simulink model "IEEE34_PMSG"  (R2024a)
settings: Solver=FixedStepDiscrete  StartTime=0.0  StopTime=ttotal  RelTol=1e-3
values from neighbouring files (symbols this model uses):
  C0_300 = 4.9597e-09    [Data_input_DFIG.mat]    (also in Data_input_PMSG.mat)
  C0_301 = 4.8339e-09    [Data_input_DFIG.mat]    (also in Data_input_PMSG.mat)
  C1_300 = 1.0146e-08    [Data_input_DFIG.mat]    (also in Data_input_PMSG.mat)
  C1_301 = 9.7319e-09    [Data_input_DFIG.mat]    (also in Data_input_PMSG.mat)
  CC = [20000 9000 135000 20000 150000 10000 16000 7000 105000 16000 75000 5000 ... (36 elements, 6x6)]    [Data_input_DFIG.mat]    (also in Data_input_PMSG.mat)
  CD = [0 0 34000 135000 0 0 0 7000 0 7000 2000 4000 ... (114 elements, 19x6)]    [Data_input_DFIG.mat]    (also in Data_input_PMSG.mat)
  cte = 1e-06    [Data_input_DFIG.mat]    (also in Data_input_PMSG.mat)
  L0_300 = 0.0039    [Data_input_DFIG.mat]    (also in Data_input_PMSG.mat)
  L0_301 = 0.0043    [Data_input_DFIG.mat]    (also in Data_input_PMSG.mat)
  L1_300 = 0.0014    [Data_input_DFIG.mat]    (also in Data_input_PMSG.mat)
  L1_301 = 0.0014    [Data_input_DFIG.mat]    (also in Data_input_PMSG.mat)
  R0_300 = 1.0909    [Data_input_DFIG.mat]    (also in Data_input_PMSG.mat)
  R0_301 = 1.4885    [Data_input_DFIG.mat]    (also in Data_input_PMSG.mat)
  R1_300 = 0.6983    [Data_input_DFIG.mat]    (also in Data_input_PMSG.mat)
  R1_301 = 1.0537    [Data_input_DFIG.mat]    (also in Data_input_PMSG.mat)
  tf_AB = 1.75    [Data_input_DFIG.mat]    (also in Data_input_PMSG.mat = 2.65)
  tf_ABC = 1.75    [Data_input_DFIG.mat]    (also in Data_input_PMSG.mat = 2.65)
  tf_ABT = 1.75    [Data_input_DFIG.mat]    (also in Data_input_PMSG.mat = 2.65)
  tf_AT = 1.75    [Data_input_DFIG.mat]    (also in Data_input_PMSG.mat = 2.65)
  tf_BC = 1.75    [Data_input_DFIG.mat]    (also in Data_input_PMSG.mat = 2.65)
  tf_BCT = 1.75    [Data_input_DFIG.mat]    (also in Data_input_PMSG.mat = 2.65)
  tf_BT = 1.75    [Data_input_DFIG.mat]    (also in Data_input_PMSG.mat = 2.65)
  tf_CA = 1.75    [Data_input_DFIG.mat]    (also in Data_input_PMSG.mat = 2.65)
  tf_CAT = 1.75    [Data_input_DFIG.mat]    (also in Data_input_PMSG.mat = 2.65)
  tf_CT = 1.75    [Data_input_DFIG.mat]    (also in Data_input_PMSG.mat = 2.65)
  Ts = 5.008e-06    [Data_input_DFIG.mat]    (also in Data_input_PMSG.mat = 1.0016e-05)
undefined symbols (not defined in the file or in its folder): D1, Delta, DiscIntNeverNeededParam, find_system
libraries: spsThreePhaseSeriesRLCLoadLib x31, spsThreePhasePISectionLineLib x22, spsGroundLib x15, spsSeriesRLCLoadLib x14, spsThreePhaseFaultLib x10, spsSecondOrderFilterLib x9, spsPiSectionLineLib x8, spsThreePhaseVIMeasurementLib x6, spsabctodq0Lib x5, simulink_extras x4, spsFirstOrderFilterLib x4, spsThreePhaseTransformerTwoWindingsLib x3
(part 1 of 4)
settings Model: Creator=hani  LastModifiedBy=jucar
settings SolverCC: AlgebraicLoopSolver=TrustRegion
settings DataIOCC: LimitDataPoints=on  SaveFormat=Array  SignalLoggingSaveFormat=ModelDataLogs  ReturnWorkspaceOutputs=off
settings OptimizationCC: ExpressionDepthLimit=2147483647  LifeSpan=inf
settings DebuggingCC: UnderspecifiedInitializationDetection=Classic  MergeDetectMultiDrivingBlocksExec=none  FcnCallInpInsideContextMsg=warning  UnconnectedInputMsg=warning  UnconnectedOutputMsg=warning  UnconnectedLineMsg=warning  StateNameClashWarn=warning  SFUnexpectedBacktrackingDiag=warning  SFNoUnconditionalDefaultTransitionDiag=warning  SFExecutionAtInitializationDiag=none  ArithmeticOperatorsInVariantConditions=warning
settings HardwareCC: ProdBitPerPointer=32  ProdBitPerSizeT=32  ProdBitPerPtrDiffT=32  ProdLargestAtomicFloat=None  ProdIntDivRoundTo=Undefined  ProdEndianess=Unspecified  ProdWordSize=32  ProdHWDeviceType=32-bit Generic
settings ModelReferenceCC: EnableRefExpFcnMdlSchedulingChecks=on  PropagateSignalLabelsOutOfModel=off
settings SFSimCC: SimUseLocalCustomCode=off  SimParseCustomCode=off  CustomCodeUndefinedFunction=UseInterfaceOnly
settings RTWCC: RTWUseLocalCustomCode=off  GPUComputeCapability=3.5
settings CodeAppCC: StateflowObjectComments=on
settings GRTTargetCC: TargetLangStandard=C89/C90 (ANSI)  CombineOutputUpdateFcns=off  GRTInterface=on
settings ConfigComp: CovMetricSettings=dw  CovSaveCumulativeToWorkspaceVar=on  CovSaveSingleToWorkspaceVar=on  CovExternalEMLEnable=off

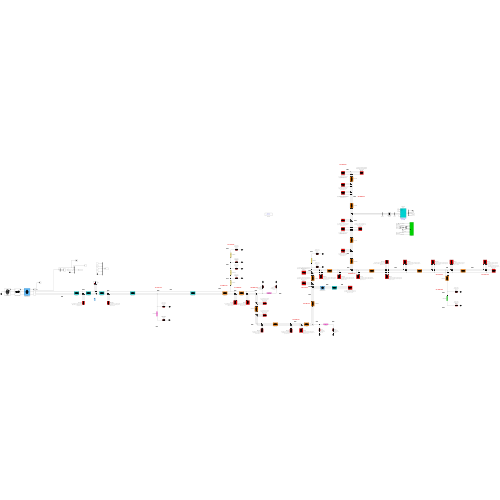
[thumbnail: Simulink's stored preview of the top-level diagram]
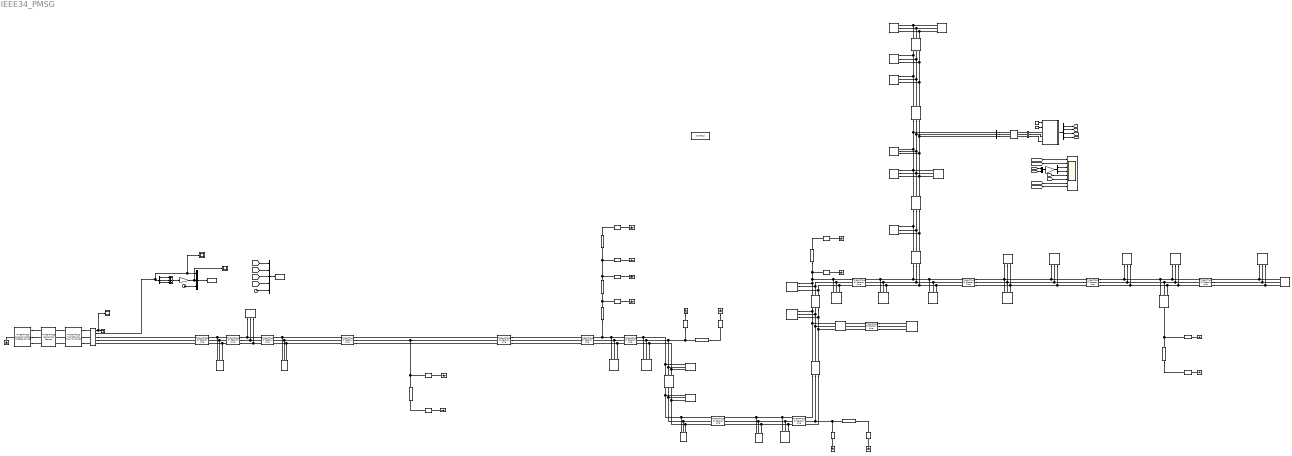
== system IEEE34_PMSG ==
  note: 806
  note: 832
  note: 862
  note: 842
  note: 808
  note: 800
  note: 826
  note: 844
  note: 850
  note: 834
  note: 830
  note: 824
  note: 848
  note: 840
  note: 838
  note: 888
  note: 854
  note: 57.5888 km
  note: 858
  note: 846
  note: 41.3247 km
  note: 864
  note: 890
  note: 816
  note: 860
  note: 856
  note: 55.9825 km
  note: 31.6291 km
  note: 57.7503 km
  note: 802
  note: 828
  note: 11.1374 km
  note: 34.8386 km
  note: 836
  note: 52.709 km
  note: 52.712 km
  note: 57.6772 km
  note: 852
  note: 1
  note: 810
  note: 820
  note: 818
  note: 51.1119 km
  note: 822
  note: 31.7266 km
  note: 57.4151 km
  note: 57.5004 km
  note: 812
  note: 10 MW Wind Farm
      | (5 x 2 MW)
  " " : spsThreePhaseVIMeasurementLib/Three-Phase V-I Measurement  VoltageMeasurement=phase-to-ground  SetLabelV=off  LabelV=Vabc  Vpu=off  VpuLL=off  CurrentMeasurement=yes  SetLabelI=off  LabelI=Iabc  Ipu=off  Pbase=100e6  Vbase=24.9e3  OutputType=Complex  PhasorSimulation=off  PSBequivalent=0
  0.0853 km : spsThreePhasePISectionLineLib/Three-Phase PI Section Line  LConnTagsString=a|b|c  RConnTagsString=A|B|C  Length=0.0853  Frequency=60  Resistances=[ R1_301 R0_301]  Inductances=[ L1_301 L0_301]  Capacitances=[C1_301 C0_301]
  0.0853 km1 : spsThreePhasePISectionLineLib/Three-Phase PI Section Line  LConnTagsString=a|b|c  RConnTagsString=A|B|C  Length=0.0853  Frequency=60  Resistances=[ R1_301 R0_301]  Inductances=[ L1_301 L0_301]  Capacitances=[C1_301 C0_301]
  0.0975 km : spsThreePhasePISectionLineLib/Three-Phase PI Section Line  LConnTagsString=a|b|c  RConnTagsString=A|B|C  Length=0.0975  Frequency=60  Resistances=[ R1_301 R0_301]  Inductances=[ L1_301 L0_301]  Capacitances=[C1_301 C0_301]
  0.1585 km : spsThreePhasePISectionLineLib/Three-Phase PI Section Line  LConnTagsString=a|b|c  RConnTagsString=A|B|C  Length=0.1585  Frequency=60  Resistances=[ R1_301 R0_301]  Inductances=[ L1_301 L0_301]  Capacitances=[C1_301 C0_301]
  0.1615 km : spsThreePhasePISectionLineLib/Three-Phase PI Section Line  LConnTagsString=a|b|c  RConnTagsString=A|B|C  Length=0.1615  Frequency=60  Resistances=[ R1_301 R0_301]  Inductances=[ L1_301 L0_301]  Capacitances=[C1_301 C0_301]
  0.2136 km : spsThreePhasePISectionLineLib/Three-Phase PI Section Line  LConnTagsString=a|b|c  RConnTagsString=A|B|C  Length=0.2136  Frequency=60  Resistances=[ R1_300 R0_300]  Inductances=[ L1_300 L0_300]  Capacitances=[C1_300 C0_300]
  0.2560 km : spsThreePhasePISectionLineLib/Three-Phase PI Section Line  LConnTagsString=a|b|c  RConnTagsString=A|B|C  Length=0.2560  Frequency=60  Resistances=[ R1_301 R0_301]  Inductances=[ L1_301 L0_301]  Capacitances=[C1_301 C0_301]
  0.2621 km : spsThreePhasePISectionLineLib/Three-Phase PI Section Line  LConnTagsString=a|b|c  RConnTagsString=A|B|C  Length=0.2621  Frequency=60  Resistances=[ R1_301 R0_301]  Inductances=[ L1_301 L0_301]  Capacitances=[C1_301 C0_301]
  0.3137 km : spsThreePhasePISectionLineLib/Three-Phase PI Section Line  LConnTagsString=a|b|c  RConnTagsString=A|B|C  Length=0.3137  Frequency=60  Resistances=[ R1_300 R0_300]  Inductances=[ L1_300 L0_300]  Capacitances=[C1_300 C0_300]
  0.4115 km : spsThreePhasePISectionLineLib/Three-Phase PI Section Line  LConnTagsString=a|b|c  RConnTagsString=A|B|C  Length=0.4115  Frequency=60  Resistances=[ R1_301 R0_301]  Inductances=[ L1_301 L0_301]  Capacitances=[C1_301 C0_301]
  0.4938 Km : spsPiSectionLineLib/Pi Section Line  LConnTagsString=__new0  RConnTagsString=__new0  Phases=1  PiSections=1  Length=0.4938  Frequency=60  Resistance=1.7395  Inductance=2.4e-3  Capacitance=6.964e-9  SpecifyConductance=off  Conductance=0  Measurements=None  Measurements2=None
      settings: LibrarySourceBlock=sps_lib/Power Grid Elements/Pi Section Line
  0.5212 Km : spsPiSectionLineLib/Pi Section Line  LConnTagsString=__new0  RConnTagsString=__new0  Phases=1  PiSections=1  Length=0.5212  Frequency=60  Resistance=1.7395  Inductance=2.4e-3  Capacitance=6.964e-9  SpecifyConductance=off  Conductance=0  Measurements=None  Measurements2=None
      settings: LibrarySourceBlock=sps_lib/Power Grid Elements/Pi Section Line
  0.6157 km : spsThreePhasePISectionLineLib/Three-Phase PI Section Line  LConnTagsString=a|b|c  RConnTagsString=A|B|C  Length=0.6157  Frequency=60  Resistances=[ R1_301 R0_301]  Inductances=[ L1_301 L0_301]  Capacitances=[C1_301 C0_301]
  0.7864 km : spsThreePhasePISectionLineLib/Three-Phase PI Section Line  LConnTagsString=a|b|c  RConnTagsString=A|B|C  Length=0.7864  Frequency=60  Resistances=[ R1_300 R0_300]  Inductances=[ L1_300 L0_300]  Capacitances=[C1_300 C0_300]
  0.8169 km : spsThreePhasePISectionLineLib/Three-Phase PI Section Line  LConnTagsString=a|b|c  RConnTagsString=A|B|C  Length=0.8169  Frequency=60  Resistances=[ R1_301 R0_301]  Inductances=[ L1_301 L0_301]  Capacitances=[C1_301 C0_301]
  1.05*345 kV : spsThreePhaseProgrammableVoltageSourceLib/Three-Phase Programmable Voltage Source  PositiveSequence=[1.05*345e3 0 60]  VariationEntity=None  VariationType=Table of time-amplitude pairs  VariationTypeAlt=Step  VariationStep=0.2  VariationRate=10  VariationMagnitude=0.3  VariationFrequency=2  VariationTiming="[5  20]"  VariationPhaseA=off  Amplitudes="[ 1 0.95   1.1 ]"  TimeValues="[0  10 50]"  HarmonicGeneration=off  HarmonicA=[3 0.2 -25 0]  HarmonicB=[2 0.15 35 2]  Timing="[0.05  3]"  BusType=swing  Pref=0  Qref=0  Qmin=-inf  Qmax=inf
  1.1095 km : spsThreePhasePISectionLineLib/Three-Phase PI Section Line  LConnTagsString=a|b|c  RConnTagsString=A|B|C  Length=1.1095  Frequency=60  Resistances=[ R1_301 R0_301]  Inductances=[ L1_301 L0_301]  Capacitances=[C1_301 C0_301]
  1.4813 Km : spsPiSectionLineLib/Pi Section Line  LConnTagsString=__new0  RConnTagsString=__new0  Phases=1  PiSections=1  Length=1.4813  Frequency=60  Resistance=1.1941  Inductance=2.3e-3  Capacitance=7.1924e-9  SpecifyConductance=off  Conductance=0  Measurements=None  Measurements2=None
      settings: LibrarySourceBlock=sps_lib/Power Grid Elements/Pi Section Line
  1.4935 km : spsThreePhasePISectionLineLib/Three-Phase PI Section Line  LConnTagsString=a|b|c  RConnTagsString=A|B|C  Length=1.4935  Frequency=60  Resistances=[ R1_301 R0_301]  Inductances=[ L1_301 L0_301]  Capacitances=[C1_301 C0_301]
  1.7691 Km : spsPiSectionLineLib/Pi Section Line  LConnTagsString=__new0  RConnTagsString=__new0  Phases=1  PiSections=1  Length=1.7691  Frequency=60  Resistance=1.7395  Inductance=2.4e-3  Capacitance=6.964e-9  SpecifyConductance=off  Conductance=0  Measurements=None  Measurements2=None
      settings: LibrarySourceBlock=sps_lib/Power Grid Elements/Pi Section Line
  1.7691 Km1 : spsPiSectionLineLib/Pi Section Line  LConnTagsString=__new0  RConnTagsString=__new0  Phases=1  PiSections=1  Length=1.7691  Frequency=60  Resistance=1.7395  Inductance=2.4e-3  Capacitance=6.964e-9  SpecifyConductance=off  Conductance=0  Measurements=None  Measurements2=None
      settings: LibrarySourceBlock=sps_lib/Power Grid Elements/Pi Section Line
  1.7770 km : spsThreePhasePISectionLineLib/Three-Phase PI Section Line  LConnTagsString=a|b|c  RConnTagsString=A|B|C  Length=1.7770  Frequency=60  Resistances=[ R1_301 R0_301]  Inductances=[ L1_301 L0_301]  Capacitances=[C1_301 C0_301]
  11.2288 km : spsThreePhasePISectionLineLib/Three-Phase PI Section Line  LConnTagsString=a|b|c  RConnTagsString=A|B|C  Length=11.2288  Frequency=60  Resistances=[ R1_301 R0_301]  Inductances=[ L1_301 L0_301]  Capacitances=[C1_301 C0_301]
  14.6761 Km : spsPiSectionLineLib/Pi Section Line  LConnTagsString=__new0  RConnTagsString=__new0  Phases=1  PiSections=1  Length=14.6761  Frequency=60  Resistance=1.7395  Inductance=2.4e-3  Capacitance=6.964e-9  SpecifyConductance=off  Conductance=0  Measurements=None  Measurements2=None
      settings: LibrarySourceBlock=sps_lib/Power Grid Elements/Pi Section Line
  2.5 MVA 345 KV/24.9 KV : spsThreePhaseTransformerTwoWindingsLib/Three-Phase Transformer (Two Windings)  Winding1Connection=Delta (D1)  Winding2Connection=Yg  CoreType=Three single-phase transformers  SetSaturation=off  Hysteresis=off  DataFile='hysteresis'  SetInitialFlux=off  Measurements=None  UNITS=pu  NominalPower=[ 2500e3 , 60 ]  Winding1=[345e3, 0.01, 0.08 ]  Winding2=[24.9e3 , 0.01, 0.08 ]  Rm=500  Lm=500  L0=0.5  Saturation=[ 0,0 ; 0.0024,1.2 ; 1.0,1.52 ]  InitialFluxes=[ 0.8 , -0.8 , 0.7 ]  BreakLoop=off  DiscreteSolver=Trapezoidal iterative  DataType=off  TransfoNumber=1
  20.4917 km : spsThreePhasePISectionLineLib/Three-Phase PI Section Line  LConnTagsString=a|b|c  RConnTagsString=A|B|C  Length=20.4917  Frequency=60  Resistances=[ R1_300 R0_300]  Inductances=[ L1_300 L0_300]  Capacitances=[C1_300 C0_300]
  24.9 kV/ 575 V 1.25 MVA : spsThreePhaseTransformerTwoWindingsLib/Three-Phase Transformer (Two Windings)  Winding1Connection=Yg  Winding2Connection=Yg  CoreType=Three single-phase transformers  SetSaturation=off  Hysteresis=off  DataFile='hysteresis'  SetInitialFlux=off  Measurements=None  UNITS=pu  NominalPower="[1.25e6  60]"  Winding1=[24.9e3 , 0.025/30 , 0.025]  Winding2=[575, 0.025/30 , 0.025]  Rm=500  Lm=inf  L0=0.5  Saturation=[ 0,0 ; 0.0024,1.2 ; 1.0,1.52 ]  InitialFluxes=[ 0.8 , -0.8 , 0.7 ]  BreakLoop=off  DiscreteSolver=Trapezoidal iterative  DataType=off  TransfoNumber=0
  3.1120 km : spsThreePhasePISectionLineLib/Three-Phase PI Section Line  LConnTagsString=a|b|c  RConnTagsString=A|B|C  Length=3.1120  Frequency=60  Resistances=[ R1_301 R0_301]  Inductances=[ L1_301 L0_301]  Capacitances=[C1_301 C0_301]
  3.2187 km : spsThreePhasePISectionLineLib/Three-Phase PI Section Line  LConnTagsString=a|b|c  RConnTagsString=A|B|C  Length=3.2187  Frequency=60  Resistances=[ R1_300 R0_300]  Inductances=[ L1_300 L0_300]  Capacitances=[C1_300 C0_300]
  4.1880 Km : spsPiSectionLineLib/Pi Section Line  LConnTagsString=__new0  RConnTagsString=__new0  Phases=1  PiSections=1  Length=4.1880  Frequency=60  Resistance=1.7395  Inductance=2.4e-3  Capacitance=6.964e-9  SpecifyConductance=off  Conductance=0  Measurements=None  Measurements2=None
      settings: LibrarySourceBlock=sps_lib/Power Grid Elements/Pi Section Line
  500 kVA 24.9 KV/4.16 KV : spsThreePhaseTransformerTwoWindingsLib/Three-Phase Transformer (Two Windings)  Winding1Connection=Yg  Winding2Connection=Yg  CoreType=Three single-phase transformers  SetSaturation=off  Hysteresis=off  DataFile='hysteresis'  SetInitialFlux=off  Measurements=None  UNITS=pu  NominalPower=[ 500e3 , 60 ]  Winding1=[24.9e3 , 0.019 , 0.0408 ]  Winding2=[ 4.16e3 , 0.019 , 0.0408 ]  Rm=500  Lm=500  L0=0.5  Saturation=[ 0,0 ; 0.0024,1.2 ; 1.0,1.52 ]  InitialFluxes=[ 0.8 , -0.8 , 0.7 ]  BreakLoop=off  DiscreteSolver=Trapezoidal iterative  DataType=off  TransfoNumber=1
  6.2301 km : spsThreePhasePISectionLineLib/Three-Phase PI Section Line  LConnTagsString=a|b|c  RConnTagsString=A|B|C  Length=6.2301  Frequency=60  Resistances=[ R1_301 R0_301]  Inductances=[ L1_301 L0_301]  Capacitances=[C1_301 C0_301]
  7.1110 Km : spsPiSectionLineLib/Pi Section Line  LConnTagsString=__new0  RConnTagsString=__new0  Phases=1  PiSections=1  Length=7.1110  Frequency=60  Resistance=1.7395  Inductance=2.4e-3  Capacitance=6.964e-9  SpecifyConductance=off  Conductance=0  Measurements=None  Measurements2=None
      settings: LibrarySourceBlock=sps_lib/Power Grid Elements/Pi Section Line
  802 Yg-PQ : spsThreePhaseSeriesRLCLoadLib/Three-Phase Series RLC Load  LConnTagsString=A|B|C  Configuration=Y (grounded)  NominalVoltage=120e3  Vabc=[ 1.04738 1.04828 1.0485]*14376  Vabcp=[1e3 1e3 1e3]  NominalFrequency=60  UnbalancedPower=on  ActivePower=1e+006  InductivePower=0  CapacitivePower=0  Pabc="[cte CD(1,3)  CD(1,5)]/2"  QLabc=[0 CD(1,4) CD(1,6)]/2  QCabc=[0 0 0]  Pabcp=[10e3 9e3 11e3]  QLabcp=[100 90 110]  QCabcp=[100 90 110]  Measurements=None  LoadType=constant PQ
      settings: AttributesFormatString=|
      | P= %<Pabc> W
      | Ql=%<QLabc> var
      | Qc=%<QCabc> var
  806 Yg-PQ : spsThreePhaseSeriesRLCLoadLib/Three-Phase Series RLC Load  LConnTagsString=A|B|C  Configuration=Y (grounded)  NominalVoltage=120e3  Vabc=[ 1.04562 1.04717 1.04753]*14376  Vabcp=[1e3 1e3 1e3]  NominalFrequency=60  UnbalancedPower=on  ActivePower=1e+006  InductivePower=0  CapacitivePower=0  Pabc="[cte CD(1,3)  CD(1,5)]/2"  QLabc=[0 CD(1,4) CD(1,6)]/2  QCabc=[0 0 0]  Pabcp=[10e3 9e3 11e3]  QLabcp=[100 90 110]  QCabcp=[100 90 110]  Measurements=None  LoadType=constant PQ
      settings: AttributesFormatString=|
      | P= %<Pabc> W
      | Ql=%<QLabc> var
      | Qc=%<QCabc> var
  808-I : spsSeriesRLCLoadLib/Series RLC Load  LConnTagsString=a  RConnTagsString=__new0  NominalVoltage=1.01367*14376  NominalFrequency=60  ActivePower=CD(2,3)/2  InductivePower=CD(2,4)/2  CapacitivePower=0  Setx0=off  InitialVoltage=0  SetiL0=off  InitialCurrent=0  Measurements=None  LoadType=constant I
      settings: AttributesFormatString=|
      | P=%<ActivePower> W
      | Ql=%<InductivePower> var
      | Qc=%<CapacitivePower> var
  810-I : spsSeriesRLCLoadLib/Series RLC Load  LConnTagsString=a  RConnTagsString=__new0  NominalVoltage=1.0136*14376  NominalFrequency=60  ActivePower=CD(2,3)/2  InductivePower=CD(2,4)/2  CapacitivePower=0  Setx0=off  InitialVoltage=0  SetiL0=off  InitialCurrent=0  Measurements=None  LoadType=constant I
      settings: AttributesFormatString=|
      | P=%<ActivePower> W
      | Ql=%<InductivePower> var
      | Qc=%<CapacitivePower> var
  816 D-I : spsThreePhaseSeriesRLCLoadLib/Three-Phase Series RLC Load  LConnTagsString=A|B|C  Configuration=Delta  NominalVoltage=120e3  Vabc="[1  1  1]*120e3/sqrt(3)"  Vabcp=[ 1.74036 1.75352 1.73649]*14376  NominalFrequency=60  UnbalancedPower=on  ActivePower=1e+006  InductivePower=0  CapacitivePower=0  Pabc="[17 66  117]*1e3/2"  QLabc="[10 38  68]*1e3/2"  QCabc=[0 0 0]  Pabcp=[cte CD(5,3) 1e-6]/2  QLabcp=[0 CD(5,4) 0]/2  QCabcp="[0  0  0]"  Measurements=None  LoadType=constant I
      settings: AttributesFormatString=|
      | P= %<Pabcp> W
      | Ql=%<QLabcp> var
      | Qc=%<QCabcp> var
  818-Z : spsSeriesRLCLoadLib/Series RLC Load  LConnTagsString=a  RConnTagsString=__new0  NominalVoltage=14376  NominalFrequency=60  ActivePower=CD(3,1)/2  InductivePower=CD(3,2)/2  CapacitivePower=0  Setx0=off  InitialVoltage=0  SetiL0=off  InitialCurrent=0  Measurements=None  LoadType=constant Z
      settings: AttributesFormatString=|
      | P=%<ActivePower> W
      | Ql=%<InductivePower> var
      | Qc=%<CapacitivePower> var
  820-PQ : spsSeriesRLCLoadLib/Series RLC Load  LConnTagsString=a  RConnTagsString=__new0  NominalVoltage=0.951596*14376  NominalFrequency=60  ActivePower=CD(4,1)/2  InductivePower=CD(4,2)/2  CapacitivePower=0  Setx0=off  InitialVoltage=0  SetiL0=off  InitialCurrent=0  Measurements=None  LoadType=constant PQ
      settings: AttributesFormatString=|
      | P=%<ActivePower> W
      | Ql=%<InductivePower> var
      | Qc=%<CapacitivePower> var
  820-Z : spsSeriesRLCLoadLib/Series RLC Load  LConnTagsString=a  RConnTagsString=__new0  NominalVoltage=14376  NominalFrequency=60  ActivePower=CD(3,1)/2  InductivePower=CD(3,2)/2  CapacitivePower=0  Setx0=off  InitialVoltage=0  SetiL0=off  InitialCurrent=0  Measurements=None  LoadType=constant Z
      settings: AttributesFormatString=|
      | P=%<ActivePower> W
      | Ql=%<InductivePower> var
      | Qc=%<CapacitivePower> var
  822-PQ : spsSeriesRLCLoadLib/Series RLC Load  LConnTagsString=a  RConnTagsString=__new0  NominalVoltage=0.948407*14376  NominalFrequency=60  ActivePower=CD(4,1)/2  InductivePower=CD(4,2)/2  CapacitivePower=0  Setx0=off  InitialVoltage=0  SetiL0=off  InitialCurrent=0  Measurements=None  LoadType=constant PQ
      settings: AttributesFormatString=|
      | P=%<ActivePower> W
      | Ql=%<InductivePower> var
      | Qc=%<CapacitivePower> var
  824 D-I : spsThreePhaseSeriesRLCLoadLib/Three-Phase Series RLC Load  LConnTagsString=A|B|C  Configuration=Delta  NominalVoltage=120e3  Vabc="[1  1  1]*120e3/sqrt(3)"  Vabcp=[ 1.73284 1.74583 1.7283]*14376  NominalFrequency=60  UnbalancedPower=on  ActivePower=1e+006  InductivePower=0  CapacitivePower=0  Pabc="[17 66  117]*1e3/2"  QLabc="[10 38  68]*1e3/2"  QCabc=[0 0 0]  Pabcp="[cte  CD(5,3) 1e-6]/2"  QLabcp=[0 CD(5,4) 0]/2  QCabcp="[0  0  0]"  Measurements=None  LoadType=constant I
      settings: AttributesFormatString=|
      | P= %<Pabcp> W
      | Ql=%<QLabcp> var
      | Qc=%<QCabcp> var
  824 Yg-PQ : spsThreePhaseSeriesRLCLoadLib/Three-Phase Series RLC Load  LConnTagsString=A|B|C  Configuration=Y (grounded)  NominalVoltage=120e3  Vabc=[ 0.967979 1.01934 1.02531]*14376  Vabcp=[1e3 1e3 1e3]  NominalFrequency=60  UnbalancedPower=on  ActivePower=1e+006  InductivePower=0  CapacitivePower=0  Pabc="[cte cte  CD(7,5)]/2"  QLabc=[0 0 CD(7,6)]/2  QCabc=[0 0 0]  Pabcp=[10e3 9e3 11e3]  QLabcp=[100 90 110]  QCabcp=[100 90 110]  Measurements=None  LoadType=constant PQ
      settings: AttributesFormatString=|
      | P= %<Pabc> W
      | Ql=%<QLabc> var
      | Qc=%<QCabc> var
  824-i : spsSeriesRLCLoadLib/Series RLC Load  LConnTagsString=a  RConnTagsString=__new0  NominalVoltage=1.00963*14376  NominalFrequency=60  ActivePower=CD(6,3)/2  InductivePower=CD(6,4)/2  CapacitivePower=0  Setx0=off  InitialVoltage=0  SetiL0=off  InitialCurrent=0  Measurements=None  LoadType=constant I
      settings: AttributesFormatString=|
      | P=%<ActivePower> W
      | Ql=%<InductivePower> var
      | Qc=%<CapacitivePower> var
  826-I : spsSeriesRLCLoadLib/Series RLC Load  LConnTagsString=a  RConnTagsString=__new0  NominalVoltage=1.00953*14376  NominalFrequency=60  ActivePower=CD(6,3)/2  InductivePower=CD(6,4)/2  CapacitivePower=0  Setx0=off  InitialVoltage=0  SetiL0=off  InitialCurrent=0  Measurements=None  LoadType=constant I
      settings: AttributesFormatString=|
      | P=%<ActivePower> W
      | Ql=%<InductivePower> var
      | Qc=%<CapacitivePower> var
  828 Yg-PQ : spsThreePhaseSeriesRLCLoadLib/Three-Phase Series RLC Load  LConnTagsString=A|B|C  Configuration=Y (grounded)  NominalVoltage=120e3  Vabc=[ 0.967227 1.01863 1.02462]*14376  Vabcp=[1e3 1e3 1e3]  NominalFrequency=60  UnbalancedPower=on  ActivePower=1e+006  InductivePower=0  CapacitivePower=0  Pabc="[cte cte  CD(7,5)]/2"  QLabc=[0 0 CD(7,6)]/2  QCabc=[0 0 0]  Pabcp=[10e3 9e3 11e3]  QLabcp=[100 90 110]  QCabcp=[100 90 110]  Measurements=None  LoadType=constant PQ
      settings: AttributesFormatString=|
      | P= %<Pabc> W
      | Ql=%<QLabc> var
      | Qc=%<QCabc> var
  828 Yg-pq : spsThreePhaseSeriesRLCLoadLib/Three-Phase Series RLC Load  LConnTagsString=A|B|C  Configuration=Y (grounded)  NominalVoltage=120e3  Vabc=[ 0.967227 1.01863 1.02462]*14376  Vabcp=[1e3 1e3 1e3]  NominalFrequency=60  UnbalancedPower=on  ActivePower=1e+006  InductivePower=0  CapacitivePower=0  Pabc=[CD(8,1) cte cte]/2  QLabc=[CD(8,2) 0 0]/2  QCabc=[0 0 0]  Pabcp=[10e3 9e3 11e3]  QLabcp=[100 90 110]  QCabcp=[100 90 110]  Measurements=Branch voltages and currents  LoadType=constant PQ
      settings: AttributesFormatString=|
      | P= %<Pabc> W
      | Ql=%<QLabc> var
      | Qc=%<QCabc> var
  830 D-Z : spsThreePhaseSeriesRLCLoadLib/Three-Phase Series RLC Load  LConnTagsString=A|B|C  Configuration=Delta  NominalVoltage=120e3  Vabc="[1  1  1]*120e3/sqrt(3)"  Vabcp=[1 1 1]*24900  NominalFrequency=60  UnbalancedPower=on  ActivePower=1e+006  InductivePower=0  CapacitivePower=0  Pabc="[17 66  117]*1e3/2"  QLabc="[10 38  68]*1e3/2"  QCabc=[0 0 0]  Pabcp=[CC(6,1) CC(6,3) CC(6,5)]  QLabcp=[CC(6,2) CC(6,4) CC(6,6)]  QCabcp="[0  0  0]"  Measurements=None  LoadType=constant Z
      settings: AttributesFormatString=|
      | P= %<Pabcp> W
      | Ql=%<QLabcp> var
      | Qc=%<QCabcp> var
  830 Yg-pq : spsThreePhaseSeriesRLCLoadLib/Three-Phase Series RLC Load  LConnTagsString=A|B|C  Configuration=Y (grounded)  NominalVoltage=120e3  Vabc=[ 0.949048 1.00123 1.0079]*14376  Vabcp=[1e3 1e3 1e3]  NominalFrequency=60  UnbalancedPower=on  ActivePower=1e+006  InductivePower=0  CapacitivePower=0  Pabc=[CD(8,1) cte cte]/2  QLabc=[CD(8,2) 0 0]/2  QCabc=[0 0 0]  Pabcp=[10e3 9e3 11e3]  QLabcp=[100 90 110]  QCabcp=[100 90 110]  Measurements=None  LoadType=constant PQ
      settings: AttributesFormatString=|
      | P= %<Pabc> W
      | Ql=%<QLabc> var
      | Qc=%<QCabc> var
  832 D-Z : spsThreePhaseSeriesRLCLoadLib/Three-Phase Series RLC Load  LConnTagsString=A|B|C  Configuration=Delta  NominalVoltage=120e3  Vabc="[1  1  1]*120e3/sqrt(3)"  Vabcp=[1 1 1]*24900  NominalFrequency=60  UnbalancedPower=on  ActivePower=1e+006  InductivePower=0  CapacitivePower=0  Pabc="[17 66  117]*1e3/2"  QLabc="[10 38  68]*1e3/2"  QCabc=[0 0 0]  Pabcp=[CD(10,1) CD(10,3) CD(10,5)]/2  QLabcp=[CD(10,2) CD(10,4) CD(10,6)]/2  QCabcp="[0  0  0]"  Measurements=None  LoadType=constant Z
      settings: AttributesFormatString=|
      | P= %<Pabcp> W
      | Ql=%<QLabcp> var
      | Qc=%<QCabcp> var
  834 D-PQ : spsThreePhaseSeriesRLCLoadLib/Three-Phase Series RLC Load  LConnTagsString=A|B|C  Configuration=Delta  NominalVoltage=120e3  Vabc="[1  1  1]*120e3/sqrt(3)"  Vabcp=[ 1.74746 1.77399 1.72558]*14376  NominalFrequency=60  UnbalancedPower=on  ActivePower=1e+006  InductivePower=0  CapacitivePower=0  Pabc="[17 66  117]*1e3/2"  QLabc="[10 38  68]*1e3/2"  QCabc=[0 0 0]  Pabcp=[CD(12,1) CD(12,3) CD(12,5)]/2  QLabcp=[CD(12,2) CD(12,4) CD(12,6)]/2  QCabcp="[0  0  0]"  Measurements=Branch voltages and currents  LoadType=constant PQ
      settings: AttributesFormatString=|
      | P= %<Pabcp> W
      | Ql=%<QLabcp> var
      | Qc=%<QCabcp> var
  834 D-Z : spsThreePhaseSeriesRLCLoadLib/Three-Phase Series RLC Load  LConnTagsString=A|B|C  Configuration=Delta  NominalVoltage=120e3  Vabc="[1  1  1]*120e3/sqrt(3)"  Vabcp=[1 1 1]*24900  NominalFrequency=60  UnbalancedPower=on  ActivePower=1e+006  InductivePower=0  CapacitivePower=0  Pabc="[17 66  117]*1e3/2"  QLabc="[10 38  68]*1e3/2"  QCabc=[0 0 0]  Pabcp=[CD(13,1) CD(13,3) CD(13,5)]/2  QLabcp=[CD(13,2) CD(13,4) CD(13,6)]/2  QCabcp="[0  0  0]"  Measurements=None  LoadType=constant Z
      settings: AttributesFormatString=|
      | P= %<Pabcp> W
      | Ql=%<QLabcp> var
      | Qc=%<QCabcp> var
  836 D-I : spsThreePhaseSeriesRLCLoadLib/Three-Phase Series RLC Load  LConnTagsString=A|B|C  Configuration=Delta  NominalVoltage=120e3  Vabc="[1  1  1]*120e3/sqrt(3)"  Vabcp=[ 1.73912 1.75229 1.72823]*14376  NominalFrequency=60  UnbalancedPower=on  ActivePower=1e+006  InductivePower=0  CapacitivePower=0  Pabc="[17 66  117]*1e3/2"  QLabc="[10 38  68]*1e3/2"  QCabc=[0 0 0]  Pabcp=[CD(15,1) CD(15,3) cte]/2  QLabcp=[CD(15,2) CD(15,4) 0]/2  QCabcp="[0  0  0]"  Measurements=None  LoadType=constant I
      settings: AttributesFormatString=|
      | P= %<Pabcp> W
      | Ql=%<QLabcp> var
      | Qc=%<QCabcp> var
  836 D-PQ : spsThreePhaseSeriesRLCLoadLib/Three-Phase Series RLC Load  LConnTagsString=A|B|C  Configuration=Delta  NominalVoltage=120e3  Vabc="[1  1  1]*120e3/sqrt(3)"  Vabcp=[ 1.74629 1.77285 1.72447]*14376  NominalFrequency=60  UnbalancedPower=on  ActivePower=1e+006  InductivePower=0  CapacitivePower=0  Pabc="[17 66  117]*1e3/2"  QLabc="[10 38  68]*1e3/2"  QCabc=[0 0 0]  Pabcp=[CD(14,1) CD(14,3) CD(14,5)]/2  QLabcp=[CD(14,2) CD(14,4) CD(14,6)]/2  QCabcp="[0  0  0]"  Measurements=Branch voltages and currents  LoadType=constant PQ
      settings: AttributesFormatString=|
      | P= %<Pabcp> W
      | Ql=%<QLabcp> var
      | Qc=%<QCabcp> var
  838-PQ : spsSeriesRLCLoadLib/Series RLC Load  LConnTagsString=a  RConnTagsString=__new0  NominalVoltage=1.02454*14376  NominalFrequency=60  ActivePower=CD(16,3)/2  InductivePower=CD(16,4)/2  CapacitivePower=0  Setx0=off  InitialVoltage=0  SetiL0=off  InitialCurrent=0  Measurements=None  LoadType=constant PQ
      settings: AttributesFormatString=|
      | P=%<ActivePower> W
      | Ql=%<InductivePower> var
      | Qc=%<CapacitivePower> var
  840 D-I : spsThreePhaseSeriesRLCLoadLib/Three-Phase Series RLC Load  LConnTagsString=A|B|C  Configuration=Delta  NominalVoltage=120e3  Vabc="[1  1  1]*120e3/sqrt(3)"  Vabcp=[ 1.73912 1.75229 1.72823]*14376  NominalFrequency=60  UnbalancedPower=on  ActivePower=1e+006  InductivePower=0  CapacitivePower=0  Pabc="[17 66  117]*1e3/2"  QLabc="[10 38  68]*1e3/2"  QCabc=[0 0 0]  Pabcp=[CD(15,1) CD(15,3) cte]/2  QLabcp=[CD(15,2) CD(15,4) 0]/2  QCabcp="[0  0  0]"  Measurements=Branch voltages and currents  LoadType=constant I
      settings: AttributesFormatString=|
      | P= %<Pabcp> W
      | Ql=%<QLabcp> var
      | Qc=%<QCabcp> var
  840 Yg-I : spsThreePhaseSeriesRLCLoadLib/Three-Phase Series RLC Load  LConnTagsString=A|B|C  Configuration=Y (grounded)  NominalVoltage=120e3  Vabc=[ 0.983782 1.01226 1.01736]*14376  Vabcp=[1e3 1e3 1e3]  NominalFrequency=60  UnbalancedPower=on  ActivePower=1e+006  InductivePower=0  CapacitivePower=0  Pabc=[CC(2,1) CC(2,3) CC(2,5)]  QLabc=[CC(2,2) CC(2,4) CC(2,6)]  QCabc=[0 0 0]  Pabcp=[10e3 9e3 11e3]  QLabcp=[100 90 110]  QCabcp=[100 90 110]  Measurements=None  LoadType=constant I
      settings: AttributesFormatString=|
      | P= %<Pabc> W
      | Ql=%<QLabc> var
      | Qc=%<QCabc> var
  842 Yg-PQ : spsThreePhaseSeriesRLCLoadLib/Three-Phase Series RLC Load  LConnTagsString=A|B|C  Configuration=Y (grounded)  NominalVoltage=120e3  Vabc=[ 0.968465 1.02546 1.03552]*14376  Vabcp=[1e3 1e3 1e3]  NominalFrequency=60  UnbalancedPower=on  ActivePower=1e+006  InductivePower=0  CapacitivePower=0  Pabc=[CD(17,1) cte cte]/2  QLabc=[CD(17,2) 0 0]/2  QCabc=[0 0 0]  Pabcp=[10e3 9e3 11e3]  QLabcp=[100 90 110]  QCabcp=[100 90 110]  Measurements=None  LoadType=constant PQ
      settings: AttributesFormatString=|
      | P= %<Pabc> W
      | Ql=%<QLabc> var
      | Qc=%<QCabc> var
  844 Yg-PQ : spsThreePhaseSeriesRLCLoadLib/Three-Phase Series RLC Load  LConnTagsString=A|B|C  Configuration=Y (grounded)  NominalVoltage=120e3  Vabc=[ 0.968242 1.02513 1.0353]*14376  Vabcp=[1e3 1e3 1e3]  NominalFrequency=60  UnbalancedPower=on  ActivePower=1e+006  InductivePower=0  CapacitivePower=0  Pabc=[CD(17,1) cte cte]/2  QLabc=[CD(17,2) 0 0]/2  QCabc=[0 0 0]  Pabcp=[10e3 9e3 11e3]  QLabcp=[100 90 110]  QCabcp=[100 90 110]  Measurements=None  LoadType=constant PQ
      settings: AttributesFormatString=|
      | P= %<Pabc> W
      | Ql=%<QLabc> var
      | Qc=%<QCabc> var
  844 Yg-Z : spsThreePhaseSeriesRLCLoadLib/Three-Phase Series RLC Load  LConnTagsString=A|B|C  Configuration=Y (grounded)  NominalVoltage=120e3  Vabc=[1 1 1]*14376  Vabcp=[1e3 1e3 1e3]  NominalFrequency=60  UnbalancedPower=on  ActivePower=1e+006  InductivePower=0  CapacitivePower=0  Pabc=[CC(3,1) CC(3,3) CC(3,5)]  QLabc=[CC(3,2) CC(3,4) CC(3,6)]  QCabc=[0 0 0]  Pabcp=[10e3 9e3 11e3]  QLabcp=[100 90 110]  QCabcp=[100 90 110]  Measurements=None  LoadType=constant Z
      settings: AttributesFormatString=|
      | P= %<Pabc> W
      | Ql=%<QLabc> var
      | Qc=%<QCabc> var
  844 Yg-pq : spsThreePhaseSeriesRLCLoadLib/Three-Phase Series RLC Load  LConnTagsString=A|B|C  Configuration=Y (grounded)  NominalVoltage=120e3  Vabc=[ 0.968242 1.02513 1.0353]*14376  Vabcp=[1e3 1e3 1e3]  NominalFrequency=60  UnbalancedPower=on  ActivePower=1e+006  InductivePower=0  CapacitivePower=0  Pabc=[cte CD(18,3) CD(18,5)]/2  QLabc=[0 CD(18,4) CD(18,6)]/2  QCabc=[0 0 0]  Pabcp=[10e3 9e3 11e3]  QLabcp=[100 90 110]  QCabcp=[100 90 110]  Measurements=None  LoadType=constant PQ
      settings: AttributesFormatString=|
      | P= %<Pabc> W
      | Ql=%<QLabc> var
      | Qc=%<QCabc> var
  846 Yg-PQ : spsThreePhaseSeriesRLCLoadLib/Three-Phase Series RLC Load  LConnTagsString=A|B|C  Configuration=Y (grounded)  NominalVoltage=120e3  Vabc=[ 0.968452 1.02513 1.03559]*14376  Vabcp=[1e3 1e3 1e3]  NominalFrequency=60  UnbalancedPower=on  ActivePower=1e+006  InductivePower=0  CapacitivePower=0  Pabc=[cte CD(19,3) cte]/2  QLabc=[0 CD(19,4) 0]/2  QCabc=[0 0 0]  Pabcp=[10e3 9e3 11e3]  QLabcp=[100 90 110]  QCabcp=[100 90 110]  Measurements=None  LoadType=constant PQ
      settings: AttributesFormatString=|
      | P= %<Pabc> W
      | Ql=%<QLabc> var
      | Qc=%<QCabc> var
  846 Yg-pq : spsThreePhaseSeriesRLCLoadLib/Three-Phase Series RLC Load  LConnTagsString=A|B|C  Configuration=Y (grounded)  NominalVoltage=120e3  Vabc=[ 0.968452 1.02513 1.03559]*14376  Vabcp=[1e3 1e3 1e3]  NominalFrequency=60  UnbalancedPower=on  ActivePower=1e+006  InductivePower=0  CapacitivePower=0  Pabc=[cte CD(18,3) CD(18,5)]/2  QLabc=[0 CD(18,4) CD(18,6)]/2  QCabc=[0 0 0]  Pabcp=[10e3 9e3 11e3]  QLabcp=[100 90 110]  QCabcp=[100 90 110]  Measurements=None  LoadType=constant PQ
      settings: AttributesFormatString=|
      | P= %<Pabc> W
      | Ql=%<QLabc> var
      | Qc=%<QCabc> var
  848 D-PQ : spsThreePhaseSeriesRLCLoadLib/Three-Phase Series RLC Load  LConnTagsString=A|B|C  Configuration=Delta  NominalVoltage=120e3  Vabc="[1  1  1]*120e3/sqrt(3)"  Vabcp=[ 1.74717 1.77374 1.72552]*14376  NominalFrequency=60  UnbalancedPower=on  ActivePower=1e+006  InductivePower=0  CapacitivePower=0  Pabc="[17 66  117]*1e3/2"  QLabc="[10 38  68]*1e3/2"  QCabc=[0 0 0]  Pabcp=[CC(4,1) CC(4,3) CC(4,5)]  QLabcp=[CC(4,2) CC(4,4) CC(4,6)]  QCabcp="[0  0  0]"  Measurements=None  LoadType=constant PQ
      settings: AttributesFormatString=|
      | P= %<Pabcp> W
      | Ql=%<QLabcp> var
      | Qc=%<QCabcp> var
  848 Yg-PQ : spsThreePhaseSeriesRLCLoadLib/Three-Phase Series RLC Load  LConnTagsString=A|B|C  Configuration=Y (grounded)  NominalVoltage=120e3  Vabc=[ 0.968481 1.02515 1.03564]*14376  Vabcp=[1e3 1e3 1e3]  NominalFrequency=60  UnbalancedPower=on  ActivePower=1e+006  InductivePower=0  CapacitivePower=0  Pabc=[cte CD(19,3) cte]/2  QLabc=[0 CD(19,4) 0]/2  QCabc=[0 0 0]  Pabcp=[10e3 9e3 11e3]  QLabcp=[100 90 110]  QCabcp=[100 90 110]  Measurements=None  LoadType=constant PQ
      settings: AttributesFormatString=|
      | P= %<Pabc> W
      | Ql=%<QLabc> var
      | Qc=%<QCabc> var
  854-PQ : spsSeriesRLCLoadLib/Series RLC Load  LConnTagsString=a  RConnTagsString=__new0  NominalVoltage=1.0008*14376  NominalFrequency=60  ActivePower=CD(9,3)/2  InductivePower=CD(9,4)/2  CapacitivePower=0  Setx0=off  InitialVoltage=0  SetiL0=off  InitialCurrent=0  Measurements=None  LoadType=constant PQ
      settings: AttributesFormatString=|
      | P=%<ActivePower> W
      | Ql=%<InductivePower> var
      | Qc=%<CapacitivePower> var
  856-PQ : spsSeriesRLCLoadLib/Series RLC Load  LConnTagsString=a  RConnTagsString=__new0  NominalVoltage=1.00071*14376  NominalFrequency=60  ActivePower=CD(9,3)/2  InductivePower=CD(9,4)/2  CapacitivePower=0  Setx0=off  InitialVoltage=0  SetiL0=off  InitialCurrent=0  Measurements=None  LoadType=constant PQ
      settings: AttributesFormatString=|
      | P=%<ActivePower> W
      | Ql=%<InductivePower> var
      | Qc=%<CapacitivePower> var
  858 D-PQ : spsThreePhaseSeriesRLCLoadLib/Three-Phase Series RLC Load  LConnTagsString=A|B|C  Configuration=Delta  NominalVoltage=120e3  Vabc="[1  1  1]*120e3/sqrt(3)"  Vabcp=[ 1.75181 1.77838 1.73059]*14376  NominalFrequency=60  UnbalancedPower=on  ActivePower=1e+006  InductivePower=0  CapacitivePower=0  Pabc="[17 66  117]*1e3/2"  QLabc="[10 38  68]*1e3/2"  QCabc=[0 0 0]  Pabcp=[CD(12,1) CD(12,3) CD(12,5)]/2  QLabcp=[CD(12,2) CD(12,4) CD(12,6)]/2  QCabcp="[0  0  0]"  Measurements=None  LoadType=constant PQ
      settings: AttributesFormatString=|
      | P= %<Pabcp> W
      | Ql=%<QLabcp> var
      | Qc=%<QCabcp> var
  858 D-Z : spsThreePhaseSeriesRLCLoadLib/Three-Phase Series RLC Load  LConnTagsString=A|B|C  Configuration=Delta  NominalVoltage=120e3  Vabc="[1  1  1]*120e3/sqrt(3)"  Vabcp=[1 1 1]*24900  NominalFrequency=60  UnbalancedPower=on  ActivePower=1e+006  InductivePower=0  CapacitivePower=0  Pabc="[17 66  117]*1e3/2"  QLabc="[10 38  68]*1e3/2"  QCabc=[0 0 0]  Pabcp=[CD(10,1) CD(10,3) CD(10,5)]/2  QLabcp=[CD(10,2) CD(10,4) CD(10,6)]/2  QCabcp="[0  0  0]"  Measurements=None  LoadType=constant Z
      settings: AttributesFormatString=|
      | P= %<Pabcp> W
      | Ql=%<QLabcp> var
      | Qc=%<QCabcp> var
  858-PQ : spsSeriesRLCLoadLib/Series RLC Load  LConnTagsString=a  RConnTagsString=__new0  NominalVoltage=0.971244*14376  NominalFrequency=60  ActivePower=CD(11,1)/2  InductivePower=CD(11,2)/2  CapacitivePower=0  Setx0=off  InitialVoltage=0  SetiL0=off  InitialCurrent=0  Measurements=None  LoadType=constant PQ
      settings: AttributesFormatString=|
      | P=%<ActivePower> W
      | Ql=%<InductivePower> var
      | Qc=%<CapacitivePower> var
  860 D-PQ : spsThreePhaseSeriesRLCLoadLib/Three-Phase Series RLC Load  LConnTagsString=A|B|C  Configuration=Delta  NominalVoltage=120e3  Vabc="[1  1  1]*120e3/sqrt(3)"  Vabcp=[ 1.74676 1.77331 1.72479]*14376  NominalFrequency=60  UnbalancedPower=on  ActivePower=1e+006  InductivePower=0  CapacitivePower=0  Pabc="[17 66  117]*1e3/2"  QLabc="[10 38  68]*1e3/2"  QCabc=[0 0 0]  Pabcp=[CD(14,1) CD(14,3) CD(14,5)]/2  QLabcp=[CD(14,2) CD(14,4) CD(14,6)]/2  QCabcp="[0  0  0]"  Measurements=None  LoadType=constant PQ
      settings: AttributesFormatString=|
      | P= %<Pabcp> W
      | Ql=%<QLabcp> var
      | Qc=%<QCabcp> var
  860 D-Z : spsThreePhaseSeriesRLCLoadLib/Three-Phase Series RLC Load  LConnTagsString=A|B|C  Configuration=Delta  NominalVoltage=120e3  Vabc="[1  1  1]*120e3/sqrt(3)"  Vabcp=[1 1 1]*24900  NominalFrequency=60  UnbalancedPower=on  ActivePower=1e+006  InductivePower=0  CapacitivePower=0  Pabc="[17 66  117]*1e3/2"  QLabc="[10 38  68]*1e3/2"  QCabc=[0 0 0]  Pabcp=[CD(13,1) CD(13,3) CD(13,5)]/2  QLabcp=[CD(13,2) CD(13,4) CD(13,6)]/2  QCabcp="[0  0  0]"  Measurements=Branch voltages and currents  LoadType=constant Z
      settings: AttributesFormatString=|
      | P= %<Pabcp> W
      | Ql=%<QLabcp> var
      | Qc=%<QCabcp> var
  860 Yg-PQ : spsThreePhaseSeriesRLCLoadLib/Three-Phase Series RLC Load  LConnTagsString=A|B|C  Configuration=Y (grounded)  NominalVoltage=120e3  Vabc=[ 0.968068 1.0251 1.0352]*14376  Vabcp=[1e3 1e3 1e3]  NominalFrequency=60  UnbalancedPower=on  ActivePower=1e+006  InductivePower=0  CapacitivePower=0  Pabc=[CC(1,1) CC(1,3) CC(1,5)]  QLabc=[CC(1,2) CC(1,4) CC(1,6)]  QCabc=[0 0 0]  Pabcp=[10e3 9e3 11e3]  QLabcp=[100 90 110]  QCabcp=[100 90 110]  Measurements=None  LoadType=constant PQ
      settings: AttributesFormatString=|
      | P= %<Pabc> W
      | Ql=%<QLabc> var
      | Qc=%<QCabc> var
  862-PQ : spsSeriesRLCLoadLib/Series RLC Load  LConnTagsString=a  RConnTagsString=__new0  NominalVoltage=1.0247*14376  NominalFrequency=60  ActivePower=CD(16,3)/2  InductivePower=CD(16,4)/2  CapacitivePower=0  Setx0=off  InitialVoltage=0  SetiL0=off  InitialCurrent=0  Measurements=None  LoadType=constant PQ
      settings: AttributesFormatString=|
      | P=%<ActivePower> W
      | Ql=%<InductivePower> var
      | Qc=%<CapacitivePower> var
  864-PQ : spsSeriesRLCLoadLib/Series RLC Load  LConnTagsString=a  RConnTagsString=__new0  NominalVoltage=0.971238*14376  NominalFrequency=60  ActivePower=CD(11,1)/2  InductivePower=CD(11,2)/2  CapacitivePower=0  Setx0=off  InitialVoltage=0  SetiL0=off  InitialCurrent=0  Measurements=None  LoadType=constant PQ
      settings: AttributesFormatString=|
      | P=%<ActivePower> W
      | Ql=%<InductivePower> var
      | Qc=%<CapacitivePower> var
  890 D-I : spsThreePhaseSeriesRLCLoadLib/Three-Phase Series RLC Load  LConnTagsString=A|B|C  Configuration=Delta  NominalVoltage=120e3  Vabc="[1  1  1]*120e3/sqrt(3)"  Vabcp=[ 1.64298 1.65375 1.62682]*2401.78  NominalFrequency=60  UnbalancedPower=on  ActivePower=1e+006  InductivePower=0  CapacitivePower=0  Pabc="[17 66  117]*1e3/2"  QLabc="[10 38  68]*1e3/2"  QCabc=[0 0 0]  Pabcp=[CC(5,1) CC(5,3) CC(5,5)]  QLabcp=[CC(5,2) CC(5,4) CC(5,6)]  QCabcp="[0  0  0]"  Measurements=None  LoadType=constant I
      settings: AttributesFormatString=|
      | P= %<Pabcp> W
      | Ql=%<QLabcp> var
      | Qc=%<QCabcp> var
  9.8237 km : spsThreePhasePISectionLineLib/Three-Phase PI Section Line  LConnTagsString=a|b|c  RConnTagsString=A|B|C  Length=9.8237  Frequency=60  Resistances=[ R1_300 R0_300]  Inductances=[ L1_300 L0_300]  Capacitances=[C1_300 C0_300]
  B25 (24.9 kV) : spsThreePhaseVIMeasurementLib/Three-Phase V-I Measurement  VoltageMeasurement=phase-to-ground  SetLabelV=on  LabelV=Vabc_B25  Vpu=on  VpuLL=off  CurrentMeasurement=yes  SetLabelI=on  LabelI=Iabc_B25  Ipu=on  Pbase=1e6  Vbase=24.9e3  OutputType=Complex  PhasorSimulation=off  PSBequivalent=0
  B575 (575 V) : spsThreePhaseVIMeasurementLib/Three-Phase V-I Measurement  VoltageMeasurement=phase-to-ground  SetLabelV=on  LabelV=Vabc_B575  Vpu=on  VpuLL=off  CurrentMeasurement=yes  SetLabelI=on  LabelI=Iabc_B575  Ipu=on  Pbase=1*1e6/0.9  Vbase=575  OutputType=Complex  PhasorSimulation=off  PSBequivalent=0
  Bus Selector : BusSelector  OutputSignals=Vdc_V,wr_pu,PQ_pu.P_pu,PQ_pu.Q_pu
  Clock1 : Clock
  Clock2 : Clock
  Constant : Constant  Value=15
  Constant1 : Constant  Value=0
  Demux : Demux  Outputs=3
  Demux2 : Demux  Outputs=2
  Falta : Subsystem
      mask Display: image('thor.gif');
  Gain : Gain  Gain=1/3
  Ground{1..11,20..23} (15 alike) : spsGroundLib/Ground  LConnTagsString=a
  MW : Gain  Gain=1*1/0.9  SaturateOnIntegerOverflow=on  OutDataTypeStr=Inherit: Same as input  ParamDataTypeStr=Inherit: Same as input
  Mux : Mux  Inputs=2
  Mux2 : Mux  Inputs=5
  Mux4 : Mux  Inputs=3
  Scc3f = 1800 MVA : spsThreePhaseSeriesRLCBranchLib/Three-Phase Series RLC Branch  LConnTagsString=A|B|C  RConnTagsString=A|B|C  BranchType=RL  Resistance=5.7632  Inductance=0.1747  Capacitance=1.0  Measurements=None
  Scope : Scope  NumInputPorts=8
  Scope1 : Scope
  Scope2 : Scope
  Scope3 : Scope
  Sum : Sum  Inputs=+++
  Terminator6 : Terminator
  To Workspace1 : ToWorkspace  VariableName=I_amos  SampleTime=-1
  To Workspace3 : ToWorkspace  VariableName=Iabc0  SampleTime=-1
      settings: Decimation=deci
  Wind Turbine Type 4 : Subsystem  LoadFcn=%find_system(gcs,'FollowLinks', 'on', 'LookUnderMasks', 'all');  mask(Wind Turbine: Model 7){Nb_wt=0.5, ShowParameters=Generator data for 1 wind turbine, nom=[2e6/0.9 730 60], Reactances=[ 1.305, 0.296, 0.252, 0.474,  0.243,  0.18 ], Time_constants=[  4.49  0.0681  0.0513  ], Resistance=0.006, mec=[0.62 0.01 1], init=[ 0  0  0  0  0  0  0  0  1 ], Vnom=575, Imax_grid_conv=1.1, RL_grid=[ 0.15 0.15/50], C_var_filter1=150e3, Vdc_nom=1100, C_DClink1=90000e-6, L_R_Boost=[0.0012     5e-3], Pmec1=2e6, wind_speed_CpMax=11, wind0=11, DisplayTurbChar=off, H_WT=4.32, Ksh=0.3, D_mutual=1.5, w_wt0=1, torque0=1, Kdc=[1.1   27.5], Ki_var_reg=0.05, Ki_volt_reg=2, Kgrid_side_cur_reg=[1  50], Kspeed=[5 1], Kboost_cur_reg=[0.025 100], Kp_pitch=15, Kcompensation=[1.5  6], Kfield=[10  20], pitch_max=27, pitch_rate=10, Ts=Ts}
      mask prompts: Nb_wt "Number of wind turbines:"; ShowParameters "Display:"; nom "Nom. power, L-L volt. and freq.: [Pn (VA), Vn (Vrms), fn (Hz)]"; Reactances "Reactances [Xd Xd' Xd'' Xq Xq'' Xl] (p.u.):"; Time_constants "Time constants [Tdo' Tdo'' Tq''] (s):"; Resistance "Resistance Rs (p.u.):"; mec "Inertia constant, friction factor, and pairs of poles: [ H(s)  F(p.u.)  p ]"; init "Initial conditions: [dw(%) th(deg) ia,ib,ic(pu) pha,phb,phc(deg) Vf(pu)]:"; Vnom "Grid-side converter nominal AC voltage (V):"; Imax_grid_conv "Grid-side converter maximum AC current (pu based on generator power and converter nominal AC voltage):"; RL_grid "Grid-side coupling inductor [ L(pu) R(pu),pu based on generator power and converter nominal AC voltage] :"; C_var_filter1 "Line filter capacitor (Q=50) (var):"; Vdc_nom "Nominal DC bus voltage (V)"; C_DClink1 "DC bus capacitor (F):"; L_R_Boost "Boost converter inductance [L(H) R(ohm)]:"; Pmec1 "Nominal mechanical output power (W):"; wind_speed_CpMax "Wind speed at nominal speed and at Cp max (must be between 6 m/s and 30 m/s) (m/s):"; wind0 "Initial wind speed (m/s):"; DisplayTurbChar "Display wind turbine power characteristics:"; H_WT "Wind turbine inertia constant H (s):"; Ksh "Shaft spring constant refer to high-speed shaft (pu of nominal mechanical torque/rad):"; D_mutual "Shaft mutual damping (pu of nominal mechanical torque/pu dw):"; w_wt0 "Turbine initial speed (pu of nominal speed):"; torque0 "Initial output torque (pu of nominal mechanical torque):"; Kdc "DC bus voltage regulator gains [Kp Ki]:"; Ki_var_reg "Grid-side converter var regulator gain [ Ki]:"; Ki_volt_reg "Grid-side converter voltage regulator gain [ Ki]:"; Kgrid_side_cur_reg "Grid-side converter current regulator gains [Kp Ki]:"; Kspeed "Speed regulator gains [Kp Ki]:"; Kboost_cur_reg "Boost inductor current regulator gains [Kp Ki]:"; Kp_pitch "Pitch controller gain [Kp]:"; Kcompensation "Pitch compensation gains [Kp Ki]:"; Kfield "Field excitation gains [Kp Ki]:"; pitch_max "Maximum pitch angle (deg):"; pitch_rate "Maximum rate of change of pitch angle (deg/s)"; Ts "Sample time (s):"
      mask help: This block implements a model of a variable speed pitch controlled wind turbine using a synchronous generator.
      mask init:
      | %Generator data
      | Pnom=nom(1)*Nb_wt;
      | Vnom_gen=nom(2);
      | Fnom=nom(3);
      | Xd=Reactances(1);
      | Xd1=Reactances(2);
      | Xd2=Reactances(3);
      | Xq=Reactances(4);
      | Xq2=Reactances(5);
      | Xl=Reactances(6);
      | Tdo1=Time_constants(1);
      | Tdo2=Time_constants(2);
      | Tq2=Time_constants(3);
      | H=mec(1);
      | F=mec(2);
      | p=mec(3);
      | 
      | % Converters data
      | L_RL=RL_grid(1);
      | R_RL=RL_grid(2);
      | L_Boost=L_R_Boost(1)/Nb_wt;
      | R_Boost=L_R_Boost(2)/Nb_wt;
      | Q_filter=50;
      | C_DClink=C_DClink1*Nb_wt;
      | C_var_filter=C_var_filter1*Nb_wt;
      | 
      | % Controller data
      | Freq_filter=10000;   %Hz
      | Zeta_filter=0.707;
      | Kp_dc=Kdc(1);
      | Ki_dc=Kdc(2);
      | Kp_grid_side_cur_reg=Kgrid_side_cur_reg(1);
      | Ki_grid_side_cur_reg=Kgrid_side_cur_reg(2);
      | Kp_speed=Kspeed(1);
      | Ki_speed=Kspeed(2);
      | Kp_boost_cur_reg=Kboost_cur_reg(1);
      | Ki_boost_cur_reg=Kboost_cur_reg(2);
      | Kp_compensation=Kcompensation(1);
      | Ki_compensation=Kcompensation(2);
      | Kp_field=Kfield(1);
      | Ki_field=Kfield(2);
      | Mod_index_max=1.1;
      | T_speed=5;      %Speed reference time constant (s)
      | Iq_ref_limit_time_constant=0.3; %(s)
      | Current_reg_output_limit=1.1;   %(pu)
      | Var_reg_output_hi_limit=1.1;    %(pu)
      | Var_reg_output_low_limit=0.9;   %(pu)
      | Pitch_time_constant=0.01;       %(s)
      | Vf_limit=10;    %Field voltage limit (pu)
      | Flux_meas_time_constant=1*(1/Fnom); %(s)
      | Freq_sawtooth=2000; %Hz, Boost converter
      | Freq_PWM=3000; %Hz, Inverter
      | Ts_snub=50e-6;  %Sample time to compute snubber resistance
      | 
      | 
      | % Turbine data
      | Pmec=Pmec1*Nb_wt;
      | c1 = 0.6450;
      | c2 = 116;
      | c3 = .4;
      | c4 = 5;
      | c5 = 21;
      | c6 = .00912;  % Set Pmin in stall condition (does not vary with wind_speed_Pmax)
      | c7 = .08;
      | c8 = .035;
      | theta=0;
      | CpMax=.5;
      | lambda_CpMax=9.9495;
      | 
      | c1_c8=[c1 c2 c3 c4 c5 c6 c7 c8];
      |   
      | 
      | %   Cp = c1*(c6*lambda + (-c4 - c3*(2.5 + theta) + c2*(1/(lambda + ...
      | %   c7*(2.5 + theta)) - c8/(1 + (2.5 + theta)^3)))/exp(c5*(1/(lambda + ...
      | %   c7*(2.5 + theta)) - c8/(1 + (2.5 + theta)^3))))
      | 
      | 
      |         %%%%%%%%%%%%%%%%%%%%%%%%%%%%%%%%%%%%%%%%%%%%%%%%%%%%%%%%%%%%%%%%%%%%%%%%%%%
      |         % Operation at Cp max
      |         %%%%%%%%%%%%%%%%%%%%%%%%%%%%%%%%%%%%%%%%%%%%%%%%%%%%%%%%%%%%%%%%%%%%%%%%%%%
      |         
      |         rated_omegar=1;
      |         omegar = rated_omegar;
      |         
      |         % Enforce boundaries on wind speed
      |         % A warning could be displayed
      |         if wind_speed_CpMax < 6
      |             wind_speed_CpMax=6;
      |             disp('Warning: Wind speed at nominal speed and at Cp max has been set to 6 m/s')
      |         end
      |         if wind_speed_CpMax > 30
      |             wind_speed_CpMax=30;
      |             disp('Warning: Wind speed at nominal speed and at Cp max has been set to 30 m/s')
      |         end
      | 
      |         K1=lambda_CpMax/omegar*wind_speed_CpMax;
      |         
      |         % Calculation of K2 needed to get P equal to the requested value at
      |         % Cp max for the requested wind speed
      |         
      |         Prated=Pmec;
      |         P_rated_omegar_theta_zero=0.75;
      |         
      |         K2 = P_rated_omegar_theta_zero*Prated/(wind_speed_CpMax^3*CpMax);
      |         
      |         K1_K2=[K1 K2];
      |         
      |         %%%%%%%%%%%%%%%%%%%%%%%%%%%%%%%%%%%%%%%%%%%%%%%%%%%%%%%%%%%%%%%%%%%%%%%%%%%
      |         % End of calculation for operation at Cp max
      |         %%%%%%%%%%%%%%%%%%%%%%%%%%%%%%%%%%%%%%%%%%%%%%%%%%%%%%%%%%%%%%%%%%%%%%%%%%%
      |         
      | 
      | %%%%%%%%%%%%%%%%%%%%%%%%%%%%%%%%%%%%%%%%%%%%%%%%%%%%%%%%%%%%%%%%%%%%%%%%%%%
      | % Plot turbine characteristics
      | %%%%%%%%%%%%%%%%%%%%%%%%%%%%%%%%%%%%%%%%%%%%%%%%%%%%%%%%%%%%%%%%%%%%%%%%%%% 
      | 
      | DisplayTurbChar=get_param(gcb,'DisplayTurbChar');
      | if strcmp(DisplayTurbChar,'on')
      |     vect_theta = 0:2:30;
      |     
      |     vect_lambda = 1:0.2:30;
      |     
      |     clear Cp;
      |     
      |     for i=1:length(vect_theta)
      |      for j=1:length(vect_lambda)
      |                 Cp(i,j) = c1*(c6*vect_lambda(j) + (-c4 - c3*(2.5 + vect_theta(i)) + c2*(1/(vect_lambda(j) + ...
      |                 c7*(2.5 + vect_theta(i))) - c8/(1 + (2.5 + vect_theta(i))^3)))/exp(c5*(1/(vect_lambda(j) + ...
      |                 c7*(2.5 + vect_theta(i))) - c8/(1 + (2.5 + vect_theta(i))^3))));
      |      end
      |     end
      | 
      |     figure(1);
      |     clf;
      |     hold on;
      | 
      |     plot(vect_lambda, Cp);
      |     axis([0, 25, 0, .6]);
      |     title('Wind Turbine Cp Characteristic (pitch angle increases by step of 2 deg.)');
      |     ylabel('Cp');
      |     set(gca,'ytick',[0 .1 .2 .3 .4 .5 .6]);
      |     xlabel('Lambda');
      |     grid on;
      |     text(10.1,0.51,'Pitch angle 0 degree');
      | 
      |     hold off
      |     
      |     % Plot of the wind turbine mechanical power output (pu) lambda and Cp
      |     % characteristics against wind speed (m/s) for a range of theta.
      |     
      |     wind_speed_range = [1,.2,30];
      |     vect_wind_speed = 1:0.2:30;
      |     
      |     clear lambda;
      |     clear Cp;
      |     clear P;
      | 
      |     for i=1:length(vect_theta)
      |         for j=1:length(vect_wind_speed)
      |             lambda(i,j) = K1*omegar/vect_wind_speed(j);
      |             Cp(i,j) = c1*(c6*lambda(i,j) + (-c4 - c3*(2.5 + vect_theta(i)) + c2*(1/(lambda(i,j) + ...
      |             c7*(2.5 + vect_theta(i))) - c8/(1 + (2.5 + vect_theta(i))^3)))/exp(c5*(1/(lambda(i,j) + ...
      |             c7*(2.5 + vect_theta(i))) - c8/(1 + (2.5 + vect_theta(i))^3))));
      |             P(i,j) = K2/Prated*vect_wind_speed(j)^3*Cp(i,j);
      |         end
      |     end
      |     
      |     
      |     figure(2);
      |     clf;
      |     hold on
      |     
      |     subplot(3,1,1);
      |     plot(vect_wind_speed, P);
      |     axis([0, 35, 0, 1.5]);
      |     title('Wind Turbine Characteristics (w = 1 pu, pitch angle increases by step of 2 deg.)');
      |     ylabel('P (pu)');
      |     set(gca,'ytick',0:.5:4);
      |     grid on;
      |     
      |     subplot(3,1,2);
      |     plot(vect_wind_speed, lambda);
      |     axis([0, 35, 0, 20]);
      |     ylabel('Lambda');
      |     grid on;
      |     
      |     subplot(3,1,3)
      |     plot(vect_wind_speed, Cp);
      |     axis([0, 35, 0, .6]);
      |     xlabel('Wind Speed (m/s)');
      |     ylabel('Cp');
      |     set(gca,'ytick',[0 .1 .2 .3 .4 .5 .6]);
      |     grid on;
      | 
      |     hold off
      |     set_param(gcb,'DisplayTurbChar','off')
      |     
      | end
      mask TypeOptions ShowParameters: Generator data for 1 wind turbine | Converters data for 1 wind turbine | Turbine data for 1 wind turbine | Drive train data for 1 wind turbine | Control parameters for 1 wind turbine
      mask Callback ShowParameters:
      | BlockName=getfullname(gcb);
      | %
      | Param_Show=get_param(BlockName,'ShowParameters');
      | Param_DisplayTurbChar=get_param(BlockName,'DisplayTurbChar');
      | 
      | p_mask{3}='off';p_mask{4}='off';p_mask{5}='off';
      | p_mask{6}='off';p_mask{7}='off';p_mask{8}='off';p_mask{9}='off';
      | p_mask{10}='off';p_mask{11}='off';p_mask{12}='off';p_mask{13}='off';
      | p_mask{14}='off';p_mask{15}='off';p_mask{16}='off';p_mask{17}='off';
      | p_mask{18}='off';p_mask{19}='off';p_mask{20}='off';p_mask{21}='off';
      | p_mask{22}='off';p_mask{23}='off';p_mask{24}='off';p_mask{25}='off';
      | p_mask{26}='off';p_mask{27}='off';p_mask{28}='off';p_mask{29}='off';
      | p_mask{30}='off';p_mask{31}='off';p_mask{32}='off';p_mask{33}='off';
      | p_mask{34}='off';p_mask{35}='off';
      | 
      | switch Param_Show
      | 	case 'Generator data for 1 wind turbine'
      | 		p_mask{3}='on';p_mask{4}='on';p_mask{5}='on';
      |         p_mask{6}='on';p_mask{7}='on';p_mask{8}='on';
      |     case 'Converters data for 1 wind turbine'
      | 		p_mask{9}='on';p_mask{10}='on';p_mask{11}='on';
      |         p_mask{12}='on';p_mask{13}='on';p_mask{14}='on';p_mask{15}='on';
      | 	case 'Turbine data for 1 wind turbine'
      | 		p_mask{16}='on';p_mask{17}='on';p_mask{18}='on';p_mask{19}='on';
      |     case 'Drive train data for 1 wind turbine'
      |         p_mask{20}='on';p_mask{21}='on';p_mask{22}='on';p_mask{23}='on';
      |         p_mask{24}='on';
      |     case 'Control parameters for 1 wind turbine'
      |         p_mask{25}='on';p_mask{26}='on';p_mask{27}='on';
      |         p_mask{28}='on';p_mask{29}='on';p_mask{30}='on';p_mask{31}='on';
      |         p_mask{32}='on';p_mask{33}='on';p_mask{34}='on';p_mask{35}='on';
      | end
      | 
      | ParVisible={'on','on',p_mask{3},p_mask{4},p_mask{5},p_mask{6},...
      |     p_mask{7},p_mask{8},p_mask{9},p_mask{10},p_mask{11},p_mask{12},...
      |     p_mask{13},p_mask{14},p_mask{15},p_mask{16},p_mask{17},p_mask{18},...
      |     p_mask{19},p_mask{20},p_mask{21},p_mask{22},p_mask{23},p_mask{24},...
      |     p_mask{25},p_mask{26},p_mask{27},p_mask{28},p_mask{29},p_mask{30},...
      |     p_mask{31},p_mask{32},p_mask{33},p_mask{34},p_mask{35},'on'};
      | %
      | set_param(BlockName,'MaskVisibilities',ParVisible);
      | set_param(BlockName,'DisplayTurbChar',Param_DisplayTurbChar);
      mask Display: disp(' ');
  powergui : spspowerguiLib/powergui  SimulationMode=Discrete  SampleTime=Ts  frequency=60  Iterations=50  frequencyindice=60  Pbase=100e6  ErrMax=1e-4  UnitsV=kV  UnitsW=MW  buscounter=0  FunctionMessages=off  echomessages=off  EnableUseOfTLC=off  CurrentSourceSwitches=off  DisableSnubberDevices=off  DisableRonSwitches=off  DisableVfSwitches=off  DisplayEquations=off  AutomaticDiscreteSolvers=off  SolverType=Tustin/Backward Euler (TBE)  Interpol=off  ExternalGateDelay=off  methode=off  Ts=100  x0status=blocks  SPID=off  SwTol=0  HookPort=off  NonlinearTolerance=1e-4  nMaxIteration=100  ContinueOnMaxIteration=off  RestoreLinks=warning  ResistiveCurrentMeasurement=off  Frange=[0:2:500]  Ylog=off  Xlog=on  ShowGrid=off  save=off  variable=ZData  structure=0  ZoomFFT=on  StartTime=0.0  cycles=1  DisplayStyle=1  fundamental=60  FreqAxis=off  MaxFrequency=1000  frequencyindicesteady=1  RmsSteady=1  display=off
  wires:
  " "/2 -> Demux/1, Scope1/1, Mux4/1  "Iabc"
  [Ia] -> Mux2/1
  [Ib] -> Mux2/2
  [Ic] -> Mux2/3
  [I0] -> Mux2/4
  Mux2/1 -> To Workspace1/1
  Clock2/1 -> Mux2/5
  " "/1 -> Scope2/1, Terminator6/1  "Vabc"
  Demux/2 -> Sum/2
  Demux/1 -> Sum/1
  Demux/3 -> Sum/3
  Sum/1 -> Gain/1
  Mux4/1 -> To Workspace3/1
  Gain/1 -> Scope3/1, Mux4/2  "I0"
  Clock1/1 -> Mux4/3
  MW/1 -> Demux2/1
  [Q_pu] -> Mux/2
  Mux/1 -> MW/1
  [Vabc_B575] -> Scope/1  "Vabc_B575 (pu)"
  [Vdc] -> Scope/5  "Vdc (V)"
  [Iabc_B25] -> Scope/8  "Iabc_B25 (pu)"
  [Iabc_B575] -> Scope/2  "Iabc_B575 (pu)"
  [Vabc_B25] -> Scope/7  "Vabc_B25 (pu)"
  [P_pu] -> Mux/1
  Demux2/2 -> Scope/4  "Q (Mvar)"
  [wr] -> Scope/6  "wr (pu)"
  Demux2/1 -> Scope/3  "P (MW)"
  Bus Selector/2 -> [wr]  "<wr_pu>"
  Wind Turbine Type 4/1(m) -> Bus Selector/1
  Bus Selector/1 -> [Vdc]  "<Vdc_V>"
  Bus Selector/4 -> [Q_pu]  "<Q_pu>"
  Constant1/1 -> Wind Turbine Type 4/2(Qref_pu)
  Bus Selector/3 -> [P_pu]  "<P_pu>"
  Constant/1 -> Wind Turbine Type 4/1("Wind (m/s) ")
  connections:
  824 Yg-PQ/LConn1 -- 0.2560 km/LConn1 -- 3.1120 km/RConn1 -- 824 D-I/LConn1
  860 D-Z/LConn1 -- 0.6157 km/RConn1 -- 860 D-PQ/LConn1 -- 0.8169 km/LConn1 -- 860 Yg-PQ/LConn1
  0.8169 km/LConn2 -- 0.6157 km/RConn2 -- 860 Yg-PQ/LConn2 -- 860 D-Z/LConn2 -- 860 D-PQ/LConn2
  834 D-Z/LConn3 -- 0.6157 km/LConn3 -- 0.0853 km1/LConn3 -- 834 D-PQ/LConn3 -- 1.7770 km/RConn3
  816 D-I/LConn3 -- 0.0975 km/RConn3 -- 3.1120 km/LConn3
  830 Yg-pq/LConn3 -- 830 D-Z/LConn3 -- 0.1585 km/LConn3 -- 6.2301 km/RConn3
  1.4813 Km/RConn1 -- 838-PQ/LConn1
  834 D-Z/LConn2 -- 0.6157 km/LConn2 -- 0.0853 km1/LConn2 -- 1.7770 km/RConn2 -- 834 D-PQ/LConn2
  842 Yg-PQ/LConn2 -- 0.4115 km/LConn2 -- 0.0853 km1/RConn2
  840 D-I/LConn1 -- 840 Yg-I/LConn1 -- 0.2621 km/RConn1
  1.7770 km/LConn1 -- 858 D-Z/LConn1 -- 1.4935 km/RConn1 -- 0.4938 Km/LConn1 -- 858-PQ/LConn1 -- 858 D-PQ/LConn1
  828 Yg-pq/LConn1 -- 6.2301 km/LConn1 -- 0.2560 km/RConn1 -- 828 Yg-PQ/LConn1
  844 Yg-PQ/LConn2 -- B25 (24.9 kV)/LConn2 -- 1.1095 km/LConn2 -- 844 Yg-pq/LConn2 -- 844 Yg-Z/LConn2 -- 0.4115 km/RConn2
  830 Yg-pq/LConn1 -- 0.1585 km/LConn1 -- 830 D-Z/LConn1 -- 6.2301 km/RConn1
  0.1615 km/RConn1 -- 848 Yg-PQ/LConn1 -- 848 D-PQ/LConn1
  0.1615 km/RConn2 -- 848 Yg-PQ/LConn2 -- 848 D-PQ/LConn2
  860 D-Z/LConn3 -- 0.6157 km/RConn3 -- 860 Yg-PQ/LConn3 -- 860 D-PQ/LConn3 -- 0.8169 km/LConn3
  816 D-I/LConn1 -- 0.5212 Km/LConn1 -- 0.0975 km/RConn1 -- 3.1120 km/LConn1
  842 Yg-PQ/LConn3 -- 0.4115 km/LConn3 -- 0.0853 km1/RConn3
  858 D-PQ/LConn2 -- 1.7770 km/LConn2 -- 1.4935 km/RConn2 -- 858 D-Z/LConn2
  802 Yg-PQ/LConn3 -- 0.2136 km/LConn3 -- 0.7864 km/RConn3
  836 D-I/LConn2 -- 0.8169 km/RConn2 -- 836 D-PQ/LConn2 -- 0.0853 km/LConn2 -- 0.2621 km/LConn2
  824 Yg-PQ/LConn3 -- 0.2560 km/LConn3 -- 3.1120 km/RConn3 -- 824 D-I/LConn3
  828 Yg-pq/LConn3 -- 6.2301 km/LConn3 -- 0.2560 km/RConn3 -- 828 Yg-PQ/LConn3
  802 Yg-PQ/LConn2 -- 0.2136 km/LConn2 -- 0.7864 km/RConn2
  858 D-Z/LConn3 -- 1.7770 km/LConn3 -- 858 D-PQ/LConn3 -- 1.4935 km/RConn3
  830 D-Z/LConn2 -- 830 Yg-pq/LConn2 -- 6.2301 km/RConn2 -- 0.1585 km/LConn2
  1.7770 km/RConn1 -- 0.6157 km/LConn1 -- 834 D-Z/LConn1 -- 0.0853 km1/LConn1 -- 834 D-PQ/LConn1
  840 D-I/LConn3 -- 840 Yg-I/LConn3 -- 0.2621 km/RConn3
  842 Yg-PQ/LConn1 -- 0.4115 km/LConn1 -- 0.0853 km1/RConn1
  828 Yg-PQ/LConn2 -- 6.2301 km/LConn2 -- 828 Yg-pq/LConn2 -- 0.2560 km/RConn2
  848 D-PQ/LConn3 -- 848 Yg-PQ/LConn3 -- 0.1615 km/RConn3
  836 D-I/LConn1 -- 0.8169 km/RConn1 -- 836 D-PQ/LConn1 -- 0.0853 km/LConn1 -- 0.2621 km/LConn1
  836 D-PQ/LConn3 -- 0.8169 km/RConn3 -- 0.0853 km/LConn3 -- 0.2621 km/LConn3 -- 836 D-I/LConn3
  802 Yg-PQ/LConn1 -- 0.2136 km/LConn1 -- 0.7864 km/RConn1
  816 D-I/LConn2 -- 0.0975 km/RConn2 -- 3.1120 km/LConn2
  840 D-I/LConn2 -- 840 Yg-I/LConn2 -- 0.2621 km/RConn2
  Ground5/LConn1 -- 824-i/RConn1
  Ground10/LConn1 -- 858-PQ/RConn1
  Ground6/LConn1 -- 826-I/RConn1
  832 D-Z/LConn1 -- 1.4935 km/LConn1 -- 500 kVA 24.9 KV/4.16 KV/LConn1 -- 11.2288 km/RConn1
  832 D-Z/LConn3 -- 1.4935 km/LConn3 -- 500 kVA 24.9 KV/4.16 KV/LConn3 -- 11.2288 km/RConn3
  Ground22/LConn1 -- 862-PQ/RConn1
  Ground9/LConn1 -- 864-PQ/RConn1
  3.2187 km/LConn1 -- 500 kVA 24.9 KV/4.16 KV/RConn1
  3.2187 km/LConn3 -- 500 kVA 24.9 KV/4.16 KV/RConn3
  Ground8/LConn1 -- 856-PQ/RConn1
  864-PQ/LConn1 -- 0.4938 Km/RConn1
  1.7691 Km1/RConn1 -- 826-I/LConn1
  3.2187 km/LConn2 -- 500 kVA 24.9 KV/4.16 KV/RConn2
  Ground23/LConn1 -- 838-PQ/RConn1
  Ground7/LConn1 -- 854-PQ/RConn1
  7.1110 Km/RConn1 -- 856-PQ/LConn1
  832 D-Z/LConn2 -- 1.4935 km/LConn2 -- 500 kVA 24.9 KV/4.16 KV/LConn2 -- 11.2288 km/RConn2
  " "/RConn2 -- 0.7864 km/LConn2
  " "/RConn1 -- 0.7864 km/LConn1
  " "/RConn3 -- 0.7864 km/LConn3
  0.3137 km/RConn1 -- 9.8237 km/LConn1 -- 806 Yg-PQ/LConn1
  806 Yg-PQ/LConn2 -- 9.8237 km/LConn2 -- 0.3137 km/RConn2
  806 Yg-PQ/LConn3 -- 9.8237 km/LConn3 -- 0.3137 km/RConn3
  9.8237 km/RConn1 -- 20.4917 km/LConn1
  9.8237 km/RConn3 -- 20.4917 km/LConn3
  0.2136 km/RConn1 -- Falta/LConn1 -- 0.3137 km/LConn1
  0.2136 km/RConn2 -- Falta/LConn2 -- 0.3137 km/LConn2
  0.2136 km/RConn3 -- Falta/LConn3 -- 0.3137 km/LConn3
  11.2288 km/LConn1 -- 0.1585 km/RConn1
  11.2288 km/LConn3 -- 0.1585 km/RConn3
  7.1110 Km/LConn1 -- 854-PQ/LConn1 -- 11.2288 km/LConn2 -- 0.1585 km/RConn2
  808-I/LConn1 -- 1.7691 Km/LConn1 -- 9.8237 km/RConn2 -- 20.4917 km/LConn2
  824-i/LConn1 -- 1.7691 Km1/LConn1 -- 824 Yg-PQ/LConn2 -- 0.2560 km/LConn2 -- 3.1120 km/RConn2 -- 824 D-I/LConn2
  3.2187 km/RConn1 -- 890 D-I/LConn1
  3.2187 km/RConn2 -- 890 D-I/LConn2
  3.2187 km/RConn3 -- 890 D-I/LConn3
  1.4813 Km/LConn1 -- 862-PQ/LConn1 -- 0.0853 km/RConn2
  846 Yg-pq/LConn1 -- 1.1095 km/RConn1 -- 0.1615 km/LConn1 -- 846 Yg-PQ/LConn1
  846 Yg-pq/LConn2 -- 1.1095 km/RConn2 -- 0.1615 km/LConn2 -- 846 Yg-PQ/LConn2
  846 Yg-PQ/LConn3 -- 0.1615 km/LConn3 -- 1.1095 km/RConn3 -- 846 Yg-pq/LConn3
  Ground20/LConn1 -- 808-I/RConn1
  810-I/LConn1 -- 1.7691 Km/RConn1
  Ground1/LConn1 -- 810-I/RConn1
  4.1880 Km/LConn1 -- 820-PQ/LConn1 -- 820-Z/LConn1 -- 14.6761 Km/RConn1
  14.6761 Km/LConn1 -- 0.5212 Km/RConn1 -- 818-Z/LConn1
  Ground21/LConn1 -- 822-PQ/RConn1
  822-PQ/LConn1 -- 4.1880 Km/RConn1
  Ground3/LConn1 -- 820-Z/RConn1
  Ground4/LConn1 -- 820-PQ/RConn1
  Ground2/LConn1 -- 818-Z/RConn1
  0.4115 km/RConn1 -- 844 Yg-PQ/LConn1 -- 844 Yg-Z/LConn1 -- B25 (24.9 kV)/LConn1 -- 1.1095 km/LConn1 -- 844 Yg-pq/LConn1
  2.5 MVA 345 KV/24.9 KV/RConn1 -- " "/LConn1
  2.5 MVA 345 KV/24.9 KV/RConn2 -- " "/LConn2
  2.5 MVA 345 KV/24.9 KV/RConn3 -- " "/LConn3
  Ground11/LConn1 -- 1.05*345 kV/LConn1
  1.05*345 kV/RConn2 -- Scc3f = 1800 MVA/LConn2
  1.05*345 kV/RConn3 -- Scc3f = 1800 MVA/LConn3
  1.05*345 kV/RConn1 -- Scc3f = 1800 MVA/LConn1
  Scc3f = 1800 MVA/RConn1 -- 2.5 MVA 345 KV/24.9 KV/LConn1
  2.5 MVA 345 KV/24.9 KV/LConn2 -- Scc3f = 1800 MVA/RConn2
  2.5 MVA 345 KV/24.9 KV/LConn3 -- Scc3f = 1800 MVA/RConn3
  20.4917 km/RConn1 -- 0.0975 km/LConn1
  20.4917 km/RConn2 -- 0.0975 km/LConn2
  20.4917 km/RConn3 -- 0.0975 km/LConn3
  844 Yg-pq/LConn3 -- B25 (24.9 kV)/LConn3 -- 1.1095 km/LConn3 -- 844 Yg-Z/LConn3 -- 844 Yg-PQ/LConn3 -- 0.4115 km/RConn3
  B575 (575 V)/LConn2 -- 24.9 kV/ 575 V 1.25 MVA/RConn2
  B575 (575 V)/LConn3 -- 24.9 kV/ 575 V 1.25 MVA/RConn3
  B575 (575 V)/LConn1 -- 24.9 kV/ 575 V 1.25 MVA/RConn1
  B25 (24.9 kV)/RConn1 -- 24.9 kV/ 575 V 1.25 MVA/LConn1
  B25 (24.9 kV)/RConn2 -- 24.9 kV/ 575 V 1.25 MVA/LConn2
  B25 (24.9 kV)/RConn3 -- 24.9 kV/ 575 V 1.25 MVA/LConn3
  B575 (575 V)/RConn3 -- Wind Turbine Type 4/LConn3
  B575 (575 V)/RConn1 -- Wind Turbine Type 4/LConn1
  B575 (575 V)/RConn2 -- Wind Turbine Type 4/LConn2
